simulink model "nonfeedback_relative"  (R2020a)
settings: Solver=ode4  StartTime=0.0  StopTime=10.0  FixedStep=0.001  RelTol=1e-3
values from neighbouring files (symbols this model uses):
  c1 = 150    [model_DOF.m]    (also in model_nonfeedback.m = 7)
  c2 = 1000    [hils2.m]    (also in miniHILS_data.m = 7; model_DOF.m = 15; model_nonfeedback.m = 13)
  k1 = 180000    [hils2.m]    (also in miniHILS_data.m = 2200; model_DOF.m = 2200; model_nonfeedback.m = 2200)
  k2 = 30000    [hils2.m]    (also in miniHILS_data.m = 405; model_DOF.m = 405; model_nonfeedback.m = 405)
  m1 = 30.0    (= 30)    [hils2.m]    (also in miniHILS_data.m = 1.5; model_DOF.m = 1.5; model_nonfeedback.m = 1.5)
  m2 = 300.0    (= 300)    [hils2.m]    (also in miniHILS_data.m = 6.4; model_DOF.m = 6.4; model_nonfeedback.m = 6.4)
settings Model: Creator=Peanatsu  LastModifiedBy=Peanatsu

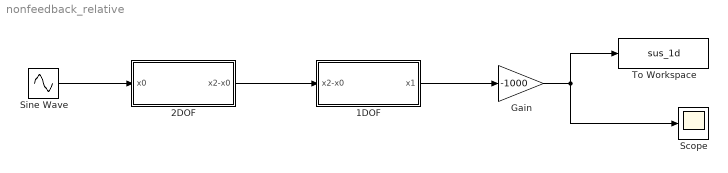
== system nonfeedback_relative ==
  1DOF : Subsystem
  2DOF : Subsystem
  Gain : Gain  Gain=-1000
  Scope : Scope
  Sine Wave : Sin  Amplitude=0.003  Frequency=2*pi  SampleTime=0
  To Workspace : ToWorkspace  VariableName=sus_1d  SaveFormat=Timeseries  SampleTime=-1
  wires:
  Gain/1 -> Scope/1, To Workspace/1
  2DOF/1(x2-x0) -> 1DOF/1(x2-x0)
  1DOF/1(x1) -> Gain/1
  Sine Wave/1 -> 2DOF/1(x0)

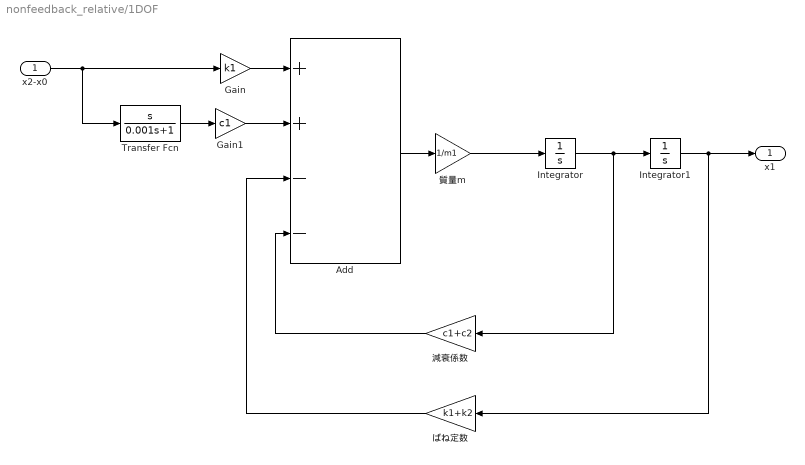
== system nonfeedback_relative/1DOF ==
  x2-x0 : Inport
  Add : Sum  Inputs=++--
  Gain : Gain  Gain=k1
  Gain1 : Gain  Gain=c1
  Integrator : Integrator
  Integrator1 : Integrator
  Transfer Fcn : TransferFcn  Numerator=[1 0]  Denominator=[0.001 1]
  "ばね定数 " : Gain  Gain=k1+k2
  減衰係数 : Gain  Gain=c1+c2
  質量m : Gain  Gain=1/m1
  x1 : Outport
  wires:
  Integrator/1 -> 減衰係数/1, Integrator1/1
  Add/1 -> 質量m/1
  x2-x0/1 -> Transfer Fcn/1, Gain/1
  質量m/1 -> Integrator/1
  Integrator1/1 -> x1/1, "ばね定数 "/1
  Gain/1 -> Add/1
  Gain1/1 -> Add/2
  Transfer Fcn/1 -> Gain1/1
  "ばね定数 "/1 -> Add/3
  減衰係数/1 -> Add/4

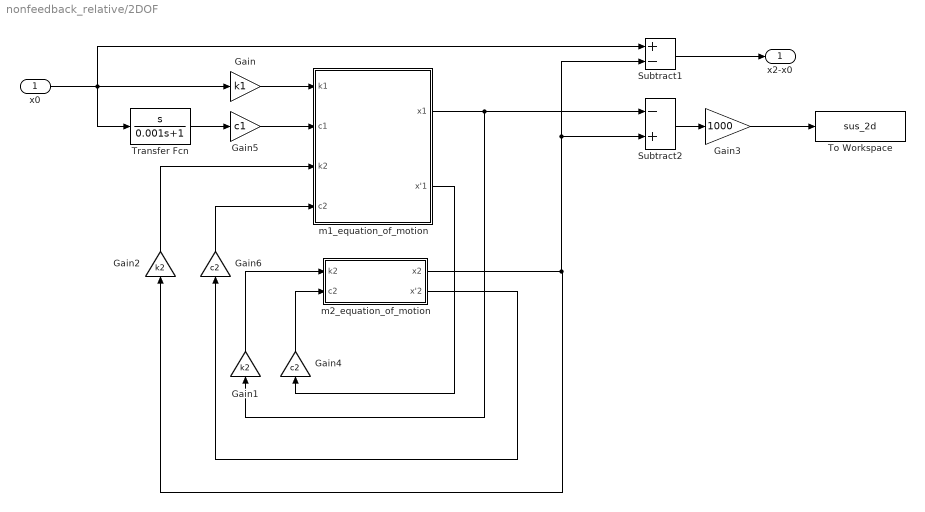
== system nonfeedback_relative/2DOF ==
  x0 : Inport
  Gain : Gain  Gain=k1
  Gain1 : Gain  Gain=k2
  Gain2 : Gain  Gain=k2
  Gain3 : Gain  Gain=1000
  Gain4 : Gain  Gain=c2
  Gain5 : Gain  Gain=c1
  Gain6 : Gain  Gain=c2
  Subtract1 : Sum  Inputs=+-
  Subtract2 : Sum  Inputs=-+
  To Workspace : ToWorkspace  VariableName=sus_2d  SaveFormat=Timeseries  SampleTime=-1
  Transfer Fcn : TransferFcn  Numerator=[1 0]  Denominator=[0.001 1]
  m1_equation_of_motion : Subsystem
  m2_equation_of_motion : Subsystem
  x2-x0 : Outport
  wires:
  x0/1 -> Transfer Fcn/1, Subtract1/1, Gain/1
  Gain/1 -> m1_equation_of_motion/1(k1)
  m1_equation_of_motion/1(x1) -> Subtract2/1, Gain1/1
  Subtract1/1 -> x2-x0/1
  Gain1/1 -> m2_equation_of_motion/1("k2 ")
  Subtract2/1 -> Gain3/1
  Gain3/1 -> To Workspace/1
  Gain2/1 -> m1_equation_of_motion/3(k2)
  Gain5/1 -> m1_equation_of_motion/2(c1)
  Transfer Fcn/1 -> Gain5/1
  m1_equation_of_motion/2(x'1) -> Gain4/1
  Gain4/1 -> m2_equation_of_motion/2(c2)
  m2_equation_of_motion/1(x2) -> Subtract1/2, Subtract2/2, Gain2/1
  m2_equation_of_motion/2(x'2) -> Gain6/1
  Gain6/1 -> m1_equation_of_motion/4(c2)

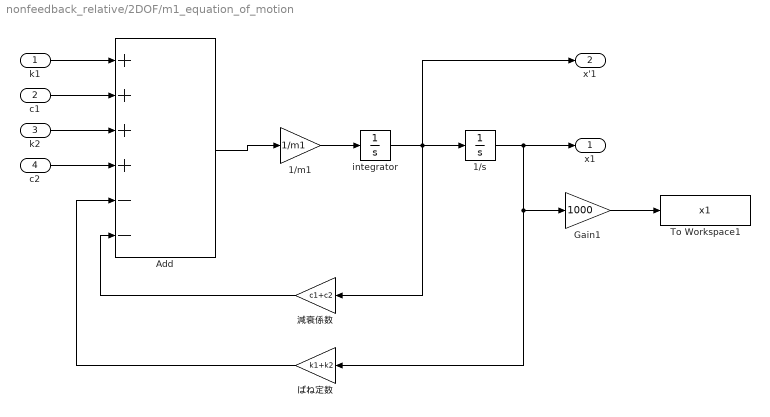
== system nonfeedback_relative/2DOF/m1_equation_of_motion ==
  k1 : Inport
  c1 : Inport  Port=2
  k2 : Inport  Port=3
  c2 : Inport  Port=4
  1/m1 : Gain  Gain=1/m1
  1/s : Integrator
  Add : Sum  Inputs=++++--
  Gain1 : Gain  Gain=1000
  To Workspace1 : ToWorkspace  VariableName=x1  SaveFormat=Timeseries  SampleTime=-1
  integrator : Integrator
  ばね定数 : Gain  Gain=k1+k2
  減衰係数 : Gain  Gain=c1+c2
  x1 : Outport
  x'1 : Outport  Port=2
  wires:
  k1/1 -> Add/1
  Add/1 -> 1/m1/1
  integrator/1 -> x'1/1, 減衰係数/1, 1/s/1
  1/s/1 -> x1/1, Gain1/1, ばね定数/1
  1/m1/1 -> integrator/1
  Gain1/1 -> To Workspace1/1
  c1/1 -> Add/2
  k2/1 -> Add/3
  減衰係数/1 -> Add/6
  ばね定数/1 -> Add/5
  c2/1 -> Add/4

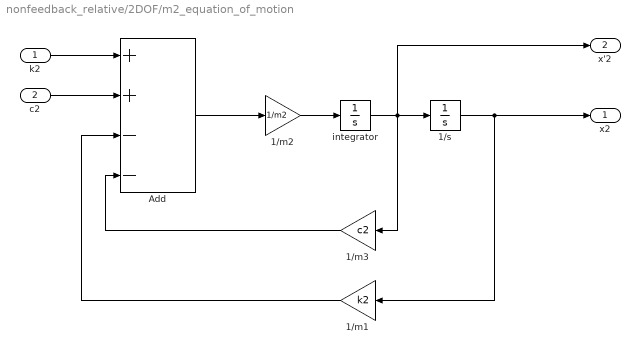
== system nonfeedback_relative/2DOF/m2_equation_of_motion ==
  "k2 " : Inport
  c2 : Inport  Port=2
  1/m1 : Gain  Gain=k2
  1/m2 : Gain  Gain=1/m2
  1/m3 : Gain  Gain=c2
  1/s : Integrator
  Add : Sum  Inputs=++--
  integrator : Integrator
  x2 : Outport
  x'2 : Outport  Port=2
  wires:
  Add/1 -> 1/m2/1
  integrator/1 -> 1/m3/1, x'2/1, 1/s/1
  1/s/1 -> 1/m1/1, x2/1
  1/m2/1 -> integrator/1
  "k2 "/1 -> Add/1
  1/m3/1 -> Add/4
  1/m1/1 -> Add/3
  c2/1 -> Add/2
